simulink model "CompareSims"  (Simulink 4.1.1)
settings: Solver=ode45  StartTime=0.0  StopTime=10.0  RelTol=1e-3
values from neighbouring files (symbols this model uses):
  ALTIAHOME = 'c:\usr\altia'    [altiahome.m]
undefined symbols (not defined in the file or in its folder): mpha, Prefix1, Prefix2
libraries: simulink3 x5
settings Model: LastModifiedBy=abrooker

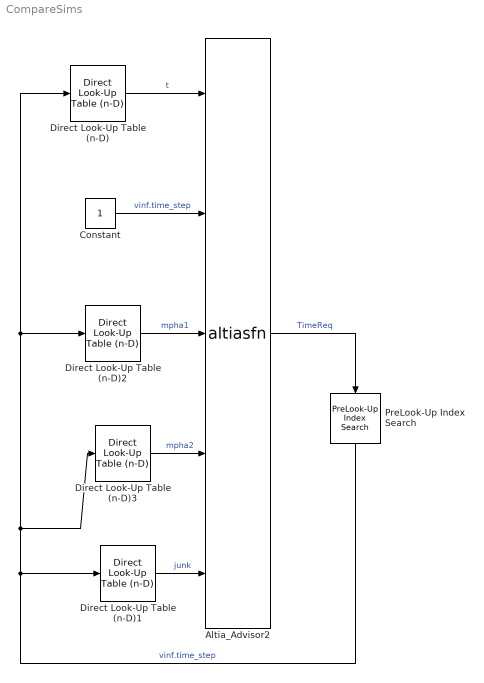
== system CompareSims ==
  Altia_Advisor2 : S-Function  FunctionName=altiasfn  Parameters=NumAltiaSfnInputs,NumAltiaSfnOutputs,ALTIAHOME  PortCounts=[]  SFunctionModules=libsdde.lib user32.lib  mask{NumAltiaSfnInputs=5, NumAltiaSfnOutputs=1}
      mask prompts: NumAltiaSfnInputs "Inputs to Altia S-Function:"; NumAltiaSfnOutputs "Outputs to Altia S-Function:"
      mask help: This block allows you to connect your signals to an Altia Design file. Specify the number of Inputs and Outputs you would like the Altia block to have (each line connected to the block can only be ONE signal wide ... no muxing into the Altia block).
      mask init:
      | altiahome
      settings: OpenFcn=AltiaClk
      mask Help: The first box is the number of inputs to the Altia S-Function.  The second box is the number of ouputs for the Altia S-Function.
      mask Display: disp('A L T I A')
  Constant : Constant  Value=1
  Direct Look-Up Table (n-D) : simulink3/Functions & Tables/Direct Look-Up Table (n-D)  maskTabDims=1  explicitNumDims=1  outDims=Element  tabIsInput=off  mxTable=mpha  clipFlag=Warning
  Direct Look-Up Table (n-D)1 : simulink3/Functions & Tables/Direct Look-Up Table (n-D)  maskTabDims=1  explicitNumDims=1  outDims=Element  tabIsInput=off  mxTable=[Prefix2,'_junk']  clipFlag=Warning
  Direct Look-Up Table (n-D)2 : simulink3/Functions & Tables/Direct Look-Up Table (n-D)  maskTabDims=1  explicitNumDims=1  outDims=Element  tabIsInput=off  mxTable=mpha  clipFlag=Warning
  Direct Look-Up Table (n-D)3 : simulink3/Functions & Tables/Direct Look-Up Table (n-D)  maskTabDims=1  explicitNumDims=1  outDims=Element  tabIsInput=off  mxTable=[Prefix1,'_mpha']  clipFlag=Warning
  PreLook-Up Index Search : simulink3/Functions & Tables/PreLook-Up Index Search  Orientation=down  bpData=[10:10:100]  searchMode=Binary Search  cacheBpFlag=off  outputFlag=on  extrapMode=Clip to Range  rangeErrorMode=None
  wires:
  Altia_Advisor2/1 -> PreLook-Up Index Search/1  "TimeReq"
  Direct Look-Up Table (n-D)/1 -> Altia_Advisor2/1  "t"
  PreLook-Up Index Search/1 -> Direct Look-Up Table (n-D)3/1, Direct Look-Up Table (n-D)2/1, Direct Look-Up Table (n-D)/1, Direct Look-Up Table (n-D)1/1  "vinf.time_step"
  Direct Look-Up Table (n-D)2/1 -> Altia_Advisor2/3  "mpha1"
  Direct Look-Up Table (n-D)3/1 -> Altia_Advisor2/4  "mpha2"
  Constant/1 -> Altia_Advisor2/2  "vinf.time_step"
  Direct Look-Up Table (n-D)1/1 -> Altia_Advisor2/5  "junk"
